simulink model "pendulo_pid_tarea"  (R2014a)
settings: Solver=ode45  StartTime=0.0  StopTime=60  MaxStep=1e-4  RelTol=1e-3
values from neighbouring files (symbols this model uses):
  b = 0.4    [TAREA_3_LABORET_MATLAB.m]
  delta = 135    [TAREA_3_LABORET_MATLAB.m]
  k1 = K(1)    [TAREA_3_LABORET_MATLAB.m]
  k2 = K(2)    [TAREA_3_LABORET_MATLAB.m]
  k3 = K(3)    [TAREA_3_LABORET_MATLAB.m]
  m = 0.1*mnom    (= 0.11)    [TAREA_3_LABORET_MATLAB.m]
settings Model: Creator=Usuario  LastModifiedBy=Ernesto
settings DataIOCC: LimitDataPoints=off  SignalLoggingSaveFormat=ModelDataLogs
settings OptimizationCC: BlockReduction=off  BooleanDataType=off  InitFltsAndDblsToZero=on
settings DebuggingCC: SaveWithParameterizedLinksMsg=none  UnderspecifiedInitializationDetection=Classic  SignalResolutionControl=TryResolveAllWithWarning  SolverPrmCheckMsg=none  MultiTaskDSMMsg=warning  MultiTaskCondExecSysMsg=none  FcnCallInpInsideContextMsg=UseLocalSettings
settings HardwareCC: TargetUnknown=on
settings RTWCC: IncludeERTFirstTime=on
settings GRTTargetCC: TargetFcnLib=ansi_tfl_tmw.mat  CombineOutputUpdateFcns=off  GRTInterface=on

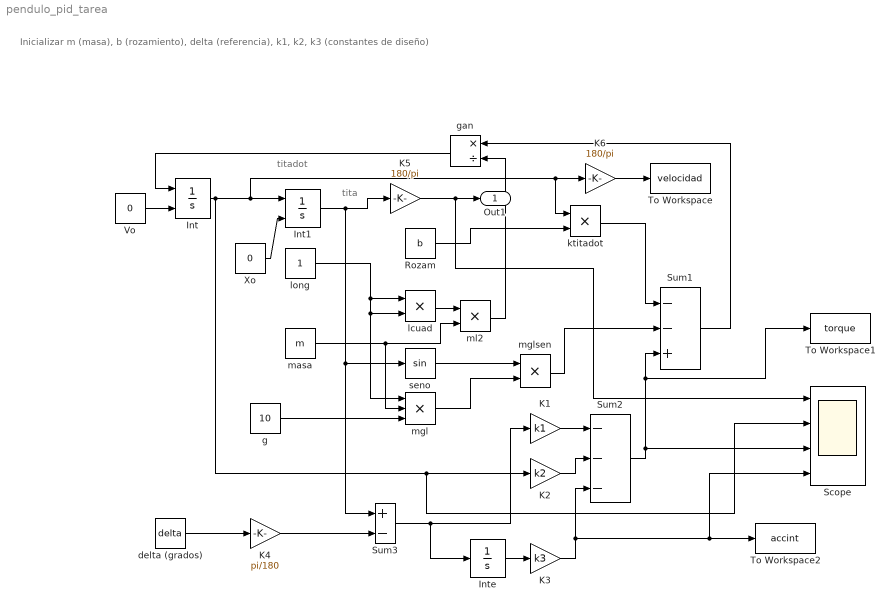
== system pendulo_pid_tarea ==
  note: Inicializar m (masa), b (rozamiento), delta (referencia), k1, k2, k3 (constantes de diseño)
  note: tita
  note: titadot
  Int : Integrator  InitialConditionSource=external  InitialCondition=-10
  Int1 : Integrator  InitialConditionSource=external  InitialCondition=2.5
  Inte : Integrator
  K1 : Gain  Gain=k1
  K2 : Gain  Gain=k2
  K3 : Gain  Gain=k3
  K4 : Gain  Gain=pi/180
  K5 : Gain  Gain=180/pi
  K6 : Gain  Gain=180/pi
  Rozam : Constant  Value=b
  Scope : Scope  NumInputPorts=4
      settings: YMin=9.5~-1.75e-07~9.5~-2.5e-08  YMax=10.5~7.5e-08~10.5~2.5e-08
  Sum1 : Sum  Inputs=--+  SaturateOnIntegerOverflow=on  InputSameDT=on  OutDataTypeStr=Inherit: Same as first input
  Sum2 : Sum  Inputs=---  SaturateOnIntegerOverflow=on  InputSameDT=on  OutDataTypeStr=Inherit: Same as first input
  Sum3 : Sum  Inputs=+-  SaturateOnIntegerOverflow=on  InputSameDT=on  OutDataTypeStr=Inherit: Same as first input
  To Workspace : ToWorkspace  VariableName=velocidad  SampleTime=-1
  To Workspace1 : ToWorkspace  VariableName=torque  SampleTime=-1
  To Workspace2 : ToWorkspace  VariableName=accint  SampleTime=-1
  Vo : Constant  Value=0
  Xo : Constant  Value=0
  delta (grados) : Constant  Value=delta
  g : Constant  Value=10
  gan : Product  Inputs=*/
  ktitadot : Product  RndMeth=Zero
  lcuad : Product  RndMeth=Zero
  long : Constant
  masa : Constant  Value=m
  mgl : Product  Inputs=3  RndMeth=Zero
  mglsen : Product  RndMeth=Zero
  ml2 : Product  RndMeth=Zero
  seno : Trigonometry
  Out1 : Outport
  wires:
  Vo/1 -> Int/2
  Xo/1 -> Int1/2
  Int/1 -> Int1/1, K6/1, ktitadot/1, Scope/2, K2/1
  long/1 -> lcuad/1, lcuad/2, mgl/1
  masa/1 -> ml2/2, mgl/2
  lcuad/1 -> ml2/1
  Rozam/1 -> ktitadot/2
  ktitadot/1 -> Sum1/1
  g/1 -> mgl/3
  K2/1 -> Sum2/2
  K1/1 -> Sum2/1
  Sum3/1 -> K1/1, Inte/1
  Sum2/1 -> Scope/3, Sum1/3, To Workspace1/1
  Int1/1 -> K5/1, Sum3/1, seno/1
  mglsen/1 -> Sum1/2
  ml2/1 -> gan/2
  gan/1 -> Int/1
  mgl/1 -> mglsen/2
  seno/1 -> mglsen/1
  Sum1/1 -> gan/1
  Inte/1 -> K3/1
  K3/1 -> Sum2/3, Scope/4, To Workspace2/1
  delta (grados)/1 -> K4/1
  K4/1 -> Sum3/2
  K6/1 -> To Workspace/1
  K5/1 -> Scope/1, Out1/1
